simulink model "EV_Model_acc"  (R2024b)
settings: Solver=ode23tb  StartTime=0  StopTime=195  RelTol=1e-3
undefined symbols (not defined in the file): Battery, BattSocInit, DiscIntNeverNeededParam, disk_abore, MotSpd, MotTrq, mu_kinetic, Ndiff, Np_Module, Ns_Module, num_pads, NumModules, RegenBrkCutOff, RegenBrkSpd_bpt, Rm
libraries: autolibshared x6, autolibsharedcoupling x3, simulink x3, mpcadaslib x1, autolibdatasheetbattery x1, autolibmappedmotor x1, autolibshareddiff x1, SignalEditorBlockLib x1
(part 1 of 3)
settings Model: SimulationMode=accelerator  Creator=mmdvn  LastModifiedBy=r
settings DebuggingCC: AlgebraicLoopMsg=none  ParameterPrecisionLossMsg=none  AllowSymbolicDim=off
settings RTWCC: GPUComputeCapability=3.5

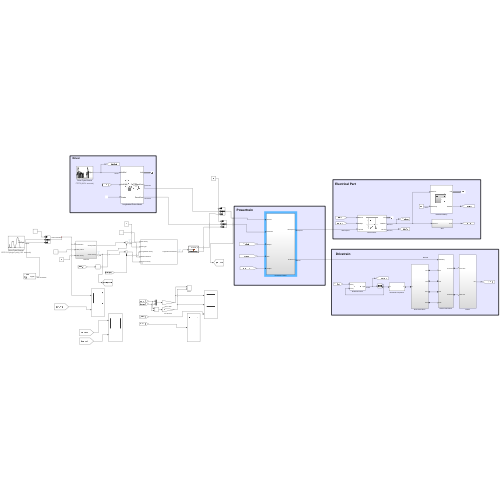
[thumbnail: Simulink's stored preview of the top-level diagram]
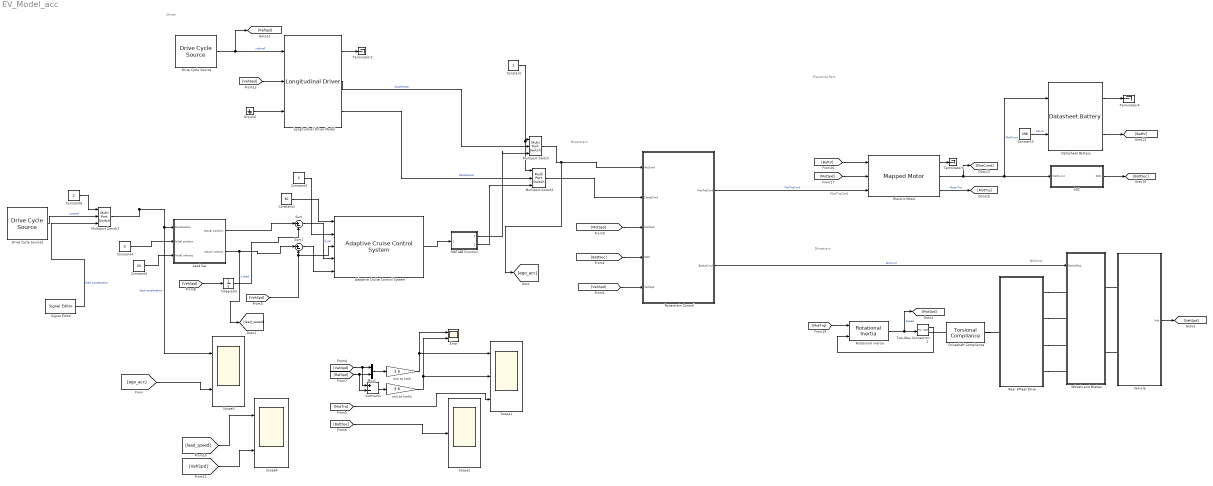
== system EV_Model_acc ==
  note: BrkCmd
  note: MotTrqCmd
  note: Drivetrain
  note: Electrical Part
  note: Powertrain
  note: Driver
  Adaptive Cruise Control System : mpcadaslib/Adaptive Cruise Control System  EgoModel=tf(1,[0.5,1,0])  InitialEgoVelocity=20  DefaultSpacing=10  MaxVelocity=50  MinAcceleration=-3  amin_ext=off  MaxAcceleration=2  amax_ext=off  Ts=0.1  PredictionHorizon=30  ControllerBehavior=0.5  suboptimal=off  maxiter=10  datatypeopt=double  optmode=off  trackmode=off
      settings: LibrarySourceBlock=mpclib/Automated Driving/Adaptive Cruise Control System
  Constant : Constant  Value=2
  Constant1 : Constant  Value=30
  Constant2 : Constant  Value=2
  Constant3 : Constant  Value=298
  Constant4 : Constant  Value=0
  Constant5 : Constant  Value=20
  Constant6 : Constant  Value=2
  Datasheet Battery : autolibdatasheetbattery/Datasheet Battery  CapacityCtrl=Parameter  OutputVlt=Unfiltered  BattChargeMax=5  Em=[2.8 3.228 3.284 3.361 3.408 3.427 3.472 3.477 3.493 3.504 3.516 3.528 3.537 3.545 3.555 3.561 3.566 3.576 3.587 3.589 3.594 3.6 3.608 3.61 3.616 3.619 3.626 3.632 3.637 3.64 3.645 3.646 3.652 3.655 3.658 3.661 3.664 3.668 3.673 3.678 3.68 3.681 3.686 3.692 3.699 3.702 3.705 3.71 3.717 3.723 3.728 3.733 3.735 3.742 3.749 3.755 3.761 3.768 3.773 3.78 3.791 3.798 3.798 3.814 3.818 3.825 3.841 3.846 3.855 3.863 3.877 3.885 3.894 3.907 3.919 3.926 3.935 3.944 3.954 3.964 3.974 3.988 3.998 4.014 4.029 4.034 4.047 4.065 4.074 4.086 4.097 4.131 4.126 4.138 4.15 4.18 4.174 4.187 4.207 4.231 4.221]  CapLUTBp=[0 0.01 0.02 0.03 0.04 0.05 0.06 0.07 0.08 0.09 0.1 0.11 0.12 0.13 0.14 0.15 0.16 0.17 0.18 0.19 0.2 0.21 0.22 0.23 0.24 0.25 0.26 0.27 0.28 0.29 0.3 0.31 0.32 0.33 0.34 0.35 0.36 0.37 0.38 0.39 0.4 0.41 0.42 0.43 0.44 0.45 0.46 0.47 0.48 0.49 0.5 0.51 0.52 0.53 0.54 0.55 0.56 0.57 0.58 0.59 0.6 0.61 0.62 0.63 0.64 0.65 0.66 0.67 0.68 0.69 0.7 0.71 0.72 0.73 0.74 0.75 0.76 0.77 0.78 0.79 0.8 0.81 0.82 0.83 0.84 0.85 0.86 0.87 0.88 0.89 0.9 0.91 0.92 0.93 0.94 0.95 0.96 0.97 0.98 0.99 1]  RInt=[0.008846 0.009319 0.009027 0.00847 0.01032 0.01314;0.006389 0.006554 0.005553 0.005525 0.006043 0.007805;0.004364 0.004101 0.00406 0.003452 0.003846 0.004517;0.002031 0.002563 0.002532 0.00246 0.002716 0.003047;0.001443 0.001825 0.001795 0.001778 0.001924 0.002234;0.0005603 0.0007192 0.0006887 0.0007557 0.0007355 0.001014;0.001028 0.001338 0.001 0.001536 0.001546 0.002789]  BattTempBp=[243.1 253.1 263.1 273.1 283.1 298.1 313.1]  CapSOCBp=[0 0.2 0.4 0.6 0.8 1]  Ns=48  Np=31  BattCapInit=3.6  Tc=1/1000  Vinit=4.221  RefBlkName='autolibdatasheetbattery/Datasheet Battery'
  Drive Cycle Source : autolibshared/Drive Cycle Source  cycleVar=FTP75  fileVar=cycleFTP75.mat  tfinal="2474  seconds"  cycleRepeat=off  outAccPort=off  outGearPort=off  gearList=No gear data  t_wot1=5  xdot_woto=0  xdot_wot1=30  t_wot2=20  xdot_wot2=0  t_wotend=30  srcUnit=m/s  outUnit=m/s  srcAccUnit=m/s/s  outAccUnit=m/s^2  dt=0  aMode=1  faultOption=off  velBnd=2  velBndUnit=mph  inUnit=m/s  timeBnd=1  failOption=off  stopSim=off  maxFaultCnt=10  maxFaultTime=2  maxTotFaultTime=15  traceOption=off  dtTrace=1  traceWindow=10  lastDCname=FTP75  lastOutUnit=mph  lastDT=0  lastTB=1  lastSB=2  forceCalcBound=off
  Drive Cycle Source1 : autolibshared/Drive Cycle Source  cycleVar=ECE R15 (single cycle)  fileVar=cycleFTP75.mat  tfinal="195  seconds"  cycleRepeat=off  outAccPort=off  outGearPort=off  gearList=No gear data  t_wot1=5  xdot_woto=0  xdot_wot1=30  t_wot2=20  xdot_wot2=0  t_wotend=30  srcUnit=m/s  outUnit=m/s  srcAccUnit=m/s/s  outAccUnit=m/s^2  dt=0  aMode=1  faultOption=off  velBnd=2  velBndUnit=mph  inUnit=m/s  timeBnd=1  failOption=off  stopSim=off  maxFaultCnt=10  maxFaultTime=2  maxTotFaultTime=15  traceOption=off  dtTrace=1  traceWindow=10  lastDCname=ECE R15 (single cycle)  lastOutUnit=mph  lastDT=0  lastTB=1  lastSB=2  forceCalcBound=off
  Driveshaft Compliance : autolibsharedcoupling/Torsional Compliance  port_config=Two-way connection  extInfo=off  k=10000  b=400  theta_o=0  domega_o=0  omega_c=100  blkID=0  aMode=1
  Electric Motor : autolibmappedmotor/Mapped Motor  w_Tmax_bp_ext=w_Tmax_bp  Tmax_w_V_ext=Tmax_w_V  w_Tmin_bp_ext=w_Tmin_bp  Tmin_w_V_ext=Tmin_w_V  port_config=Speed  param_by=Maximum torque and power  w_t=[ 0 375 750 800 ]  T_t=[0.09 0.08 0.07 0]  torque_max=450  power_max=211000  SpreadsheetTqLimitsFileName=MotorCalibrationImportData.xlsx  Tmax_w_V=[0.09 0.09 0.09;0.08 0.08 0.08;0.07 0.07 0.07;0 0 0]  w_Tmax_bp=[ 0 375 750 800 ]  V_Tmax_bp=[500 750 900]  Tmin_w_V=[-0.09 -0.09 -0.09;-0.08 -0.08 -0.08;-0.07 -0.07 -0.07;0 0 0]  w_Tmin_bp=[ 0 375 750 800 ]  V_Tmin_bp=[500 750 900]  Tc=0.02  param_loss=Tabulated efficiency data  SpreadsheetLossFileName=MotorCalibrationImportData.xlsx  SpreadsheetEffFileName=MotorCalibrationImportData.xlsx  eff=100  w_eff=375  T_eff=0.08  Piron=0  Pbase=0  w_eff_bp=[-800 -400 0 400 800]  T_eff_bp=[0 0.03 0.06 0.09]  Temp_eff_bp=[233.15 293.15 373.15]  V_eff_bp=[500 700 900]  losses_table=[1.49 1.67 2.21 3.10; 0.42 0.69 1.14 2.03; 0.06 0.24 0.78 1.68; 0.42 0.69 1.14 2.03; 1.49 1.67 2.21 3.10]  losses_table_3d=cat(3,[1.49 1.67 2.21 3.10; 0.42 0.69 1.14 2.03; 0.06 0.24 0.78 1.68; 0.42 0.69 1.14 2.03; 1.49 1.67 2.21 3.10],[1.49 1.67 2.21 3.10; 0.42 0.69 1.14 2.03; 0.06 0.24 0.78 1.68; 0.42 0.69 1.14 2.03; 1.49 1.67 2.21 3.10],[1.49 1.67 2.21 3.10; 0.42 0.69 1.14 2.03; 0.06 0.24 0.78 1.68; 0.42 0.69 1.14 2.03; 1.49 1.67 2.21 3.10])  losses_table_4d=cat(4,cat(3,[1.5645 0.441 0.063 0.441 1.5645;1.7535 0.7245 0.252 0.7245 1.7535;2.3205 1.197 0.819 1.197 2.3205;3.255 2.1315 1.764 2.1315 3.255],[1.5645 0.441 0.063 0.441 1.5645;1.7535 0.7245 0.252 0.7245 1.7535;2.3205 1.197 0.819 1.197 2.3205;3.255 2.1315 1.764 2.1315 3.255],[1.5645 0.441 0.063 0.441 1.5645;1.7535 0.7245 0.252 0.7245 1.7535;2.3205 1.197 0.819 1.197 2.3205;3.255 2.1315 1.764 2.1315 3.255]),cat(3,[1.49 0.42 0.06 0.42 1.49;1.67 0.69 0.24 0.69 1.67;2.21 1.14 0.78 1.14 2.21;3.1 2.03 1.68 2.03 3.1],[1.49 0.42 0.06 0.42 1.49;1.67 0.69 0.24 0.69 1.67;2.21 1.14 0.78 1.14 2.21;3.1 2.03 1.68 2.03 3.1],[1.49 0.42 0.06 0.42 1.49;1.67 0.69 0.24 0.69 1.67;2.21 1.14 0.78 1.14 2.21;3.1 2.03 1.68 2.03 3.1]),cat(3,[1.5347 0.4326 0.0618 0.4326 1.5347;1.7201 0.7107 0.2472 0.7107 1.7201;2.2763 1.1742 0.8034 1.1742 2.2763;3.193 2.0909 1.7304 2.0909 3.193],[1.5347 0.4326 0.0618 0.4326 1.5347;1.7201 0.7107 0.2472 0.7107 1.7201;2.2763 1.1742 0.8034 1.1742 2.2763;3.193 2.0909 1.7304 2.0909 3.193],[1.5347 0.4326 0.0618 0.4326 1.5347;1.7201 0.7107 0.2472 0.7107 1.7201;2.2763 1.1742 0.8034 1.1742 2.2763;3.193 2.0909 1.7304 2.0909 3.193]))  efficiency_table=[95 95 95 95; 95 95 95 95; 95 95 95 95; 95 95 95 95; 95 95 95 95]  efficiency_table_3d=cat(3,[95 95 95 95; 95 95 95 95; 95 95 95 95; 95 95 95 95; 95 95 95 95],[95 95 95 95; 95 95 95 95; 95 95 95 95; 95 95 95 95; 95 95 95 95],[95 95 95 95; 95 95 95 95; 95 95 95 95; 95 95 95 95; 95 95 95 95])  efficiency_table_4d=cat(4,cat(3,90*ones(5,4)',90*ones(5,4)',90*ones(5,4)'),cat(3,95*ones(5,4)',95*ones(5,4)',95*ones(5,4)'),cat(3,92*ones(5,4)',92*ones(5,4)',92*ones(5,4)'))  J=5e-6  b=1e-5  omega_o=0  T_t_extended=[0 0.07 0.08 0.09 0.08 0.07 0]  w_t_extended=[-800 -750 -375 0 375 750 800]  KLossIron=0  KLossCopper=0  x_w_eff_vec=[-800 -400 0 400 800]  x_T_eff_vec=[-0.09 -0.06 -0.03 0 0.03 0.06 0.09]  x_tmp_eff_vec=[-0.09 -0.06 -0.03 0 0.03 0.06 0.09]  x_V_eff_vec=[500 700 900]  x_losses_mat=[3.78947368421052 2.52631578947368 1.26315789473684 0 1.2 2.4 3.6;1.89473684210526 1.26315789473684 0.63157894736842 0 0.599999999999999 1.2 1.8;0 0 0 0 0 0 0;1.8 1.2 0.599999999999999 0 0.63157894736842 1.26315789473684 1.89473684210526;3.6 2.4 1.2 0 1.26315789473684 2.52631578947368 3.78947368421052]  x_losses_mat_3d=[37.8947368421052 25.2631578947368 12.6315789473684 0 12 24 36;18.9473684210526 12.6315789473684 6.3157894736842 0 5.99999999999999 12 18;0 0 0 0 0 0 0;18 12 5.99999999999999 0 6.3157894736842 12.6315789473684 18.9473684210526;36 24 12 0 12.6315789473684 25.2631578947368 37.8947368421052]  x_losses_mat_4d=cat(4,cat(3,[1.5645 0.441 0.063 0.441 1.5645;1.7535 0.7245 0.252 0.7245 1.7535;2.3205 1.197 0.819 1.197 2.3205;3.255 2.1315 1.764 2.1315 3.255],[1.5645 0.441 0.063 0.441 1.5645;1.7535 0.7245 0.252 0.7245 1.7535;2.3205 1.197 0.819 1.197 2.3205;3.255 2.1315 1.764 2.1315 3.255],[1.5645 0.441 0.063 0.441 1.5645;1.7535 0.7245 0.252 0.7245 1.7535;2.3205 1.197 0.819 1.197 2.3205;3.255 2.1315 1.764 2.1315 3.255]),cat(3,[1.49 0.42 0.06 0.42 1.49;1.67 0.69 0.24 0.69 1.67;2.21 1.14 0.78 1.14 2.21;3.1 2.03 1.68 2.03 3.1],[1.49 0.42 0.06 0.42 1.49;1.67 0.69 0.24 0.69 1.67;2.21 1.14 0.78 1.14 2.21;3.1 2.03 1.68 2.03 3.1],[1.49 0.42 0.06 0.42 1.49;1.67 0.69 0.24 0.69 1.67;2.21 1.14 0.78 1.14 2.21;3.1 2.03 1.68 2.03 3.1]),cat(3,[1.5347 0.4326 0.0618 0.4326 1.5347;1.7201 0.7107 0.2472 0.7107 1.7201;2.2763 1.1742 0.8034 1.1742 2.2763;3.193 2.0909 1.7304 2.0909 3.193],[1.5347 0.4326 0.0618 0.4326 1.5347;1.7201 0.7107 0.2472 0.7107 1.7201;2.2763 1.1742 0.8034 1.1742 2.2763;3.193 2.0909 1.7304 2.0909 3.193],[1.5347 0.4326 0.0618 0.4326 1.5347;1.7201 0.7107 0.2472 0.7107 1.7201;2.2763 1.1742 0.8034 1.1742 2.2763;3.193 2.0909 1.7304 2.0909 3.193]))  CalLossMapData={}  CalLossWithTempMapData={}  aMode=1  RefBlkName='autolibmappedmotor/Mapped Motor'
      settings: LibrarySourceBlock=autolibemachines/Mapped Motor
  Error : Scope  NumInputPorts=2
  Ground : Ground
  Integrator : Integrator
  Lead Car : Subsystem
  Longitudinal Driver Model : autolibshared/Longitudinal Driver  extAccelOvr=off  extDecelOvr=off  extAccelHld=off  extDecelHld=off  extAccelZero=off  extDecelZero=off  cntrlType=Predictive  shftType=Reverse, Neutral, Drive  velUnits=m/s  gearOut=off  Kp=1  Ki=1  Kff=0  Kg=0  VehVelVec=[0 100]  KffVec=[.1 .1]  KpVec=[10 10]  KiVec=[5 5]  KgVec=[0 0]  m=1645  Kpt=450*9.04/0.324  tau=0.12  L=4  aR=30.3/3875  bR=0.21290*4.44822/0.44704  cR=0.01278*4.44822/0.44704^2  g=9.81  vnom=1  Kaw=0  tauerr=0  tauPt=2  GearInit=0  tShift=.1  pdlVec=[0.1 0.4 0.5 0.9]  upShftTbl=[-1 12.9375 26.4375 39.9375 51.18749999999999 62.4375 72.84375 83.25;-1 16.3125 29.8125 43.3125 54.5624 65.8125 76.78125 87.75;-1 19.6875 33.1875 46.68749999999999 57.9375 69.1875 80.71875 92.25;-1 33 52.5 77.25 100.5 138.75 161.875 185]  dwnShftTbl=[1 9.5625 23.0625 36.5625 47.8125 59.0625 68.90625 78.75;1 12.9375 26.4375 39.9375 51.18749999999999 62.4375 72.84375 83.25;1 16.3125 29.8125 43.3125 54.562499 65.8125 76.78125 87.75;1 19.6875 33.1875 46.68749999999999 57.9375 69.1875 80.71875 92.25]  tClutch=.5  tRev=.5  tPark=120  aMode=1  UpGearVec="[0  1  2  3  4  5  6  7]"  DownGearVec="[1  2  3  4  5  6  7  8]"
  MATLAB Function : MATLAB Function  TreatAsAtomicUnit=on
  Multiport Switch : MultiPortSwitch  Inputs=2  SaturateOnIntegerOverflow=off  InputSameDT=off
  Multiport Switch1 : MultiPortSwitch  Inputs=2  SaturateOnIntegerOverflow=off  InputSameDT=off
  Multiport Switch2 : MultiPortSwitch  Inputs=2  SaturateOnIntegerOverflow=off  InputSameDT=off
  Mux1 : Mux  Inputs=2
  Powertrain Control : Subsystem
  Rear Wheel Drive : Subsystem  VariantControl=1
  "Rotational Inertia " : autolibsharedcoupling/Rotational Inertia  port_config=Simulink  extInfo=off  externJ=off  J=0.1  b=.001  omega_o=0  blkID=0  aMode=1
      settings: LibrarySourceBlock=autolibcoupling/Rotational Inertia
  SOC : Subsystem
  Scope1 : Scope  NumInputPorts=3
  Scope2 : Scope
  Scope3 : Scope  NumInputPorts=2
  Scope4 : Scope  NumInputPorts=2
  Signal Editor : SignalEditorBlockLib/Signal Editor  FileName=cycle.mat  ActiveScenario=Scenario  ActiveSignal=Signal 1  IsBus=off  OutputBusObjectStr=Bus: BusObject  SampleTime=0  Interpolate=off  ZeroCross=off  OutputAfterFinalValue=Setting to zero  Unit=inherit  PreserveSignalName=on  ApplySigPropsToAllScenarios=on  ApplySigPropsToAllSignals=off
  Subtract1 : Sum  Inputs=+-
  Sum : Sum  Inputs=|+-
  Sum1 : Sum  Inputs=|+-
  Terminator2 : Terminator
  Terminator3 : Terminator
  Terminator4 : Terminator
  Two-Way Connection1 : TwoWayConnection
  Vehicle : Subsystem
  Wheels and Brakes : Subsystem  VariantControl=0
  m/s to kmh : Gain  Gain=3.6
  m/s to kmh1 : Gain  Gain=3.6
  wires:
  Two-Way Connection1/1 -> "Rotational Inertia "/2
  Vehicle/1(Info) -> [VehSpd]
  [MotSpd] -> Powertrain Control/3(MotSpd)
  [BattSoc] -> Powertrain Control/4(SOC)
  Powertrain Control/1(MotTrqCmd) -> Electric Motor/3  "MotTrqCmd"
  Powertrain Control/2(BrakeCmd) -> Wheels and Brakes/1(BrakeReq)  "BrkCmd"
  Drive Cycle Source/1 -> Longitudinal Driver Model/1, [RefSpd]  "xdotref"
  Ground/1 -> Longitudinal Driver Model/3
  [VehSpd] -> Longitudinal Driver Model/2
  "Rotational Inertia "/1 -> [MotSpd], Two-Way Connection1/1  "Speed"
  Longitudinal Driver Model/2 -> Multiport Switch/2  "Accelerator"
  Longitudinal Driver Model/1 -> Terminator2/1
  [MotTrq] -> "Rotational Inertia "/1
  Constant3/1 -> Datasheet Battery/2  "Kelvin"
  [MotSpd] -> Electric Motor/2
  Datasheet Battery/1 -> Terminator4/1
  Datasheet Battery/2 -> [BattV]
  Electric Motor/3 -> [MotTrq]  "MotorTrq"
  Electric Motor/2 -> Datasheet Battery/1, SOC/1(MotCurnt), [MotCurnt]  "MotCurnt"
  Electric Motor/1 -> Terminator3/1
  SOC/1(SOC) -> [BattSoc]
  [VehSpd] -> Powertrain Control/5(VehSpd)
  [BattV] -> Electric Motor/1
  [MotTrq] -> Scope1/3
  m/s to kmh/1 -> Error/1, Scope1/1
  [RefSpd] -> Subtract1/2, Mux1/2
  [VehSpd] -> Subtract1/1, Mux1/1
  Mux1/1 -> m/s to kmh/1
  Subtract1/1 -> m/s to kmh1/1
  m/s to kmh1/1 -> Error/2, Scope1/2
  [BattSoc] -> Scope2/1
  Lead Car/1(Actual position) -> Sum/1
  Lead Car/2(Actual velocity) -> [lead_speed], Sum1/1  "v_lead"
  [VehSpd] -> Integrator/1
  [VehSpd] -> Adaptive Cruise Control System/3, Sum1/2
  Sum1/1 -> Adaptive Cruise Control System/5
  Sum/1 -> Adaptive Cruise Control System/4  "d_rel"
  Integrator/1 -> Sum/2
  Multiport Switch/1 -> [ego_acc], Powertrain Control/1(AccCmd)
  Constant/1 -> Multiport Switch1/1, Multiport Switch/1
  Adaptive Cruise Control System/1 -> MATLAB Function/1(a_desired)
  MATLAB Function/1(AccelPID_In) -> Multiport Switch/3
  Longitudinal Driver Model/3 -> Multiport Switch1/2  "Decelerator"
  Multiport Switch1/1 -> Powertrain Control/2(DecelCmd)
  MATLAB Function/2(BrakePID_In) -> Multiport Switch1/3
  Constant1/1 -> Adaptive Cruise Control System/1
  Constant2/1 -> Adaptive Cruise Control System/2
  Multiport Switch2/1 -> Scope3/1, Lead Car/1(Acceleration)  "lead acceleration"
  Constant5/1 -> Lead Car/3(Initial velocity)
  Constant4/1 -> Lead Car/2(Initial position)
  [ego_acc] -> Scope3/2
  [lead_speed] -> Scope4/1
  [VehSpd] -> Scope4/2
  Drive Cycle Source1/1 -> Multiport Switch2/2  "xdotref"
  Signal Editor/1 -> Multiport Switch2/3  "lead acceleration"
  Constant6/1 -> Multiport Switch2/1
  connections:
  Rear Wheel Drive/RConn3 -- Wheels and Brakes/LConn3
  Rear Wheel Drive/RConn4 -- Wheels and Brakes/LConn4
  Driveshaft Compliance/LConn1 -- Two-Way Connection1/RConn1
  Rear Wheel Drive/RConn1 -- Wheels and Brakes/LConn1
  Rear Wheel Drive/RConn2 -- Wheels and Brakes/LConn2
  Vehicle/LConn1 -- Wheels and Brakes/RConn1
  Vehicle/LConn2 -- Wheels and Brakes/RConn2
  Driveshaft Compliance/RConn1 -- Rear Wheel Drive/LConn1

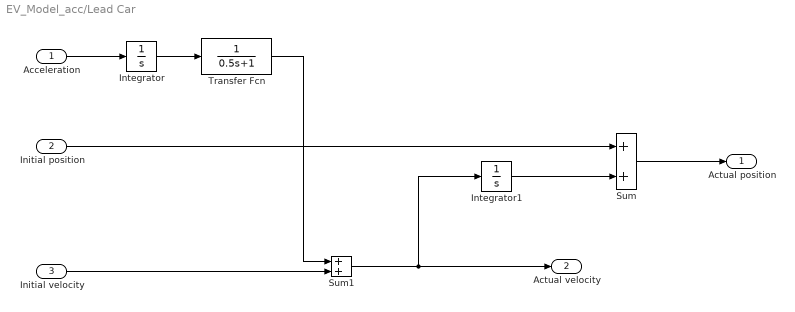
== system EV_Model_acc/Lead Car ==
  Acceleration : Inport
  Initial position : Inport  Port=2
  Initial velocity : Inport  Port=3
  Integrator : Integrator
  Integrator1 : Integrator
  Sum : Sum
  Sum1 : Sum
  Transfer Fcn : TransferFcn  Denominator=[0.5 1]
  Actual position : Outport  VectorParamsAs1DForOutWhenUnconnected=off
  Actual velocity : Outport  Port=2  VectorParamsAs1DForOutWhenUnconnected=off
  wires:
  Transfer Fcn/1 -> Sum1/1
  Initial velocity/1 -> Sum1/2
  Sum/1 -> Actual position/1
  Integrator/1 -> Transfer Fcn/1
  Sum1/1 -> Integrator1/1, Actual velocity/1
  Acceleration/1 -> Integrator/1
  Initial position/1 -> Sum/1
  Integrator1/1 -> Sum/2

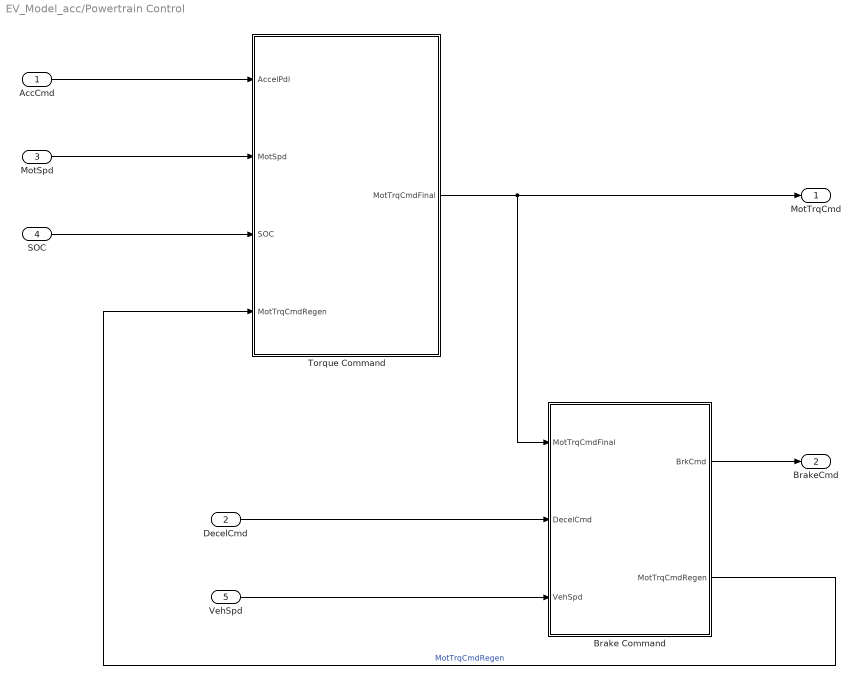
== system EV_Model_acc/Powertrain Control ==
  AccCmd : Inport
  DecelCmd : Inport  Port=2  OutDataTypeStr=double
  MotSpd : Inport  Port=3
  SOC : Inport  Port=4
  VehSpd : Inport  Port=5
  Brake Command : Subsystem  InitFcn=%[~]=autosharedicon('autolibutils',gcb,0);  VariantControl=Variant
  Torque Command : Subsystem
  MotTrqCmd : Outport  VectorParamsAs1DForOutWhenUnconnected=off
  BrakeCmd : Outport  Port=2  VectorParamsAs1DForOutWhenUnconnected=off
  wires:
  SOC/1 -> Torque Command/3(SOC)
  MotSpd/1 -> Torque Command/2(MotSpd)
  DecelCmd/1 -> Brake Command/2("DecelCmd ")
  AccCmd/1 -> Torque Command/1(AccelPdl)
  Torque Command/1(MotTrqCmdFinal) -> MotTrqCmd/1, Brake Command/1(MotTrqCmdFinal)
  Brake Command/1(" BrkCmd") -> BrakeCmd/1
  VehSpd/1 -> Brake Command/3(VehSpd)
  Brake Command/2(" MotTrqCmdRegen") -> Torque Command/4(MotTrqCmdRegen)  "MotTrqCmdRegen"

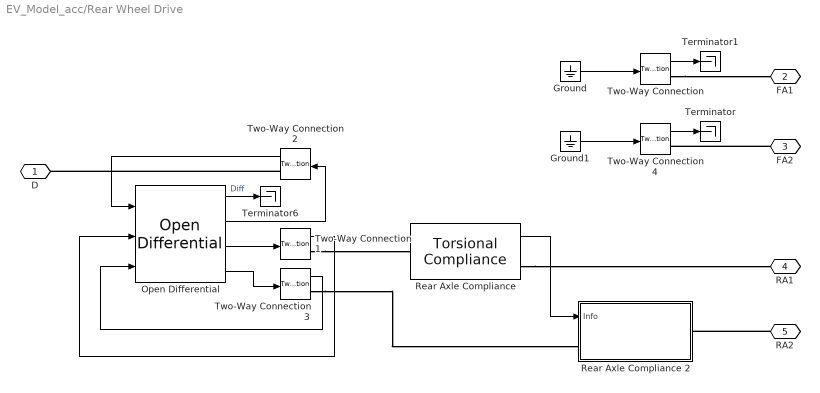
== system EV_Model_acc/Rear Wheel Drive ==
  Ground : Ground
  Ground1 : Ground
  "Open Differential " : autolibshareddiff/Open Differential  DiffEffModelPopup=Constant  InterpMethod=Linear point-slope  extTamb=off  shaftSwitchMask=To the left of center-line  Ndiff=Ndiff  Jd=0.025  bd=0.001  Jw1=0.01  bw1=0.001  Jw2=0.01  bw2=0.001  omegaw1o=0  omegaw2o=0  eta=1  eta_tbl=reshape([0.64 0.76 0.8 0.81 0.83 0.84 0.84 0.56 0.73 0.78 0.8 0.83 0.84 0.84 0.54 0.71 0.77 0.8 0.82 0.84 0.84 0.53 0.71 0.77 0.8 0.83 0.84 0.84 0.51 0.71 0.77 0.8 0.83 0.84 0.85 0.52 0.7 0.77 0.8 0.83 0.84 0.85 0.51 0.71 0.76 0.79 0.83 0.84 0.85 0.5 0.69 0.76 0.79 0.82 0.84 0.85 0.45 0.68 0.75 0.78 0.82 0.84 0.85 0.43 0.67 0.74 0.78 0.81 0.83 0.84 0.38 0.63 0.71 0.75 0.8 0.82 0.83 0.81 0.86 0.88 0.89 0.89 0.89 0.9 0.77 0.85 0.87 0.88 0.89 0.9 0.9 0.72 0.82 0.86 0.87 0.88 0.89 0.9 0.68 0.8 0.84 0.86 0.88 0.89 0.89 0.67 0.8 0.84 0.86 0.88 0.89 0.9 0.67 0.8 0.84 0.86 0.88 0.89 0.9 0.65 0.8 0.84 0.86 0.88 0.89 0.9 0.64 0.79 0.83 0.86 0.88 0.89 0.9 0.63 0.78 0.83 0.86 0.88 0.89 0.9 0.59 0.76 0.82 0.85 0.87 0.89 0.9 0.53 0.73 0.8 0.83 0.86 0.88 0.89], 7, 11, 2)  Trq_bpts=[25, 50, 75, 100, 150, 200, 250]  omega_bpts=[52.4 78.5 105 131 157 183 209 262 314 419 524]  Temp_bpts=[290 358]  Tamb=297.15  maxAbsSpd=5e3  aMode=1
      settings: LibrarySourceBlock=autolibdiff/Open Differential
  Rear Axle Compliance : autolibsharedcoupling/Torsional Compliance  port_config=Two-way connection  extInfo=on  k=10000  b=400  theta_o=0  domega_o=0  omega_c=100  blkID=0  aMode=1
  Rear Axle Compliance 2 : Subsystem
  Terminator : Terminator
  Terminator1 : Terminator
  Terminator6 : Terminator
  Two-Way Connection{,1..4} (5 alike) : TwoWayConnection
  D : PMIOPort  Side=Left
  FA1 : PMIOPort  Port=2  Side=Right
  FA2 : PMIOPort  Port=3  Side=Right
  RA1 : PMIOPort  Port=4  Side=Right
  RA2 : PMIOPort  Port=5  Side=Right
  wires:
  Two-Way Connection3/1 -> "Open Differential "/3
  "Open Differential "/4 -> Two-Way Connection3/1
  "Open Differential "/2 -> Two-Way Connection2/1
  Two-Way Connection1/1 -> "Open Differential "/2
  Two-Way Connection2/1 -> "Open Differential "/1
  "Open Differential "/1 -> Terminator6/1  "Diff"
  "Open Differential "/3 -> Two-Way Connection1/1
  Rear Axle Compliance/1 -> Rear Axle Compliance 2/1(Info)
  Two-Way Connection/1 -> Terminator1/1
  Ground/1 -> Two-Way Connection/1
  Ground1/1 -> Two-Way Connection4/1
  Two-Way Connection4/1 -> Terminator/1
  connections:
  Two-Way Connection1/RConn1 -- Rear Axle Compliance/LConn1
  Two-Way Connection3/RConn1 -- Rear Axle Compliance 2/LConn1
  Two-Way Connection2/RConn1 -- D/RConn1
  Rear Axle Compliance/RConn1 -- RA1/RConn1
  RA2/RConn1 -- Rear Axle Compliance 2/RConn1
  Two-Way Connection/RConn1 -- FA1/RConn1
  FA2/RConn1 -- Two-Way Connection4/RConn1

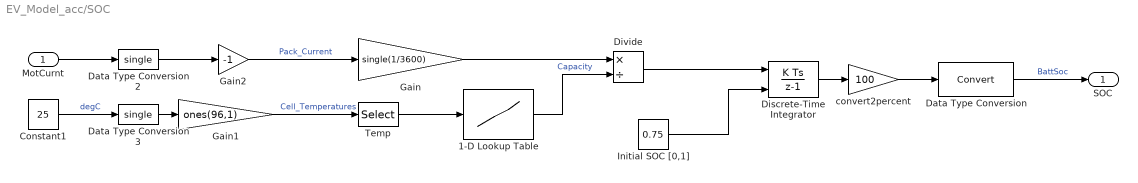
== system EV_Model_acc/SOC ==
  MotCurnt : Inport  PortDimensions=1
  1-D Lookup Table : Lookup_n-D  NumberOfTableDimensions=1  BreakpointsForDimension1=single(Battery.Temperature_LUT)  Table=single(Battery.Capacity_LUT)*Np_Module  InternalRulePriority=Speed  RndMeth=Simplest
  Constant1 : Constant  Value=25
  Data Type Conversion : DataTypeConversion  SaturateOnIntegerOverflow=off  RndMeth=Floor
  Data Type Conversion2 : DataTypeConversion  OutDataTypeStr=single  SaturateOnIntegerOverflow=off  RndMeth=Floor
  Data Type Conversion3 : DataTypeConversion  OutDataTypeStr=single  SaturateOnIntegerOverflow=off  RndMeth=Floor
  Discrete-Time Integrator : DiscreteIntegrator  InitialConditionSource=external  InitialCondition=single(BattSocInit)  SampleTime=-1  LimitOutput=on  UpperSaturationLimit=1  LowerSaturationLimit=0  ICPrevOutput=DiscIntNeverNeededParam  ICPrevScaledInput=DiscIntNeverNeededParam
  Divide : Product  Inputs=*/
  Gain : Gain  Gain=single(1/3600)
  Gain1 : Gain  Gain=ones(96,1)
  Gain2 : Gain  Gain=-1
  Initial SOC [0,1] : Constant  Value=0.75  OutDataTypeStr=single
  Temp : Selector  InputPortWidth=Ns_Module*NumModules  IndexOptions=Index vector (dialog)  Indices=1  OutputSizes=1
  convert2percent : Gain  Gain=100
  SOC : Outport
  wires:
  Gain1/1 -> Temp/1  "Cell_Temperatures"
  Gain2/1 -> Gain/1  "Pack_Current"
  Data Type Conversion2/1 -> Gain2/1
  Data Type Conversion3/1 -> Gain1/1
  MotCurnt/1 -> Data Type Conversion2/1
  Constant1/1 -> Data Type Conversion3/1  "degC"
  convert2percent/1 -> Data Type Conversion/1
  Data Type Conversion/1 -> SOC/1  "BattSoc"
  Discrete-Time Integrator/1 -> convert2percent/1
  Temp/1 -> 1-D Lookup Table/1
  Divide/1 -> Discrete-Time Integrator/1
  1-D Lookup Table/1 -> Divide/2  "Capacity"
  Gain/1 -> Divide/1
  Initial SOC [0,1]/1 -> Discrete-Time Integrator/2

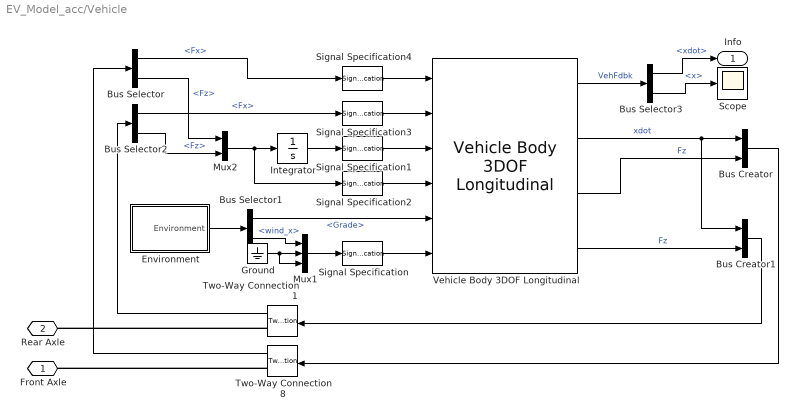
== system EV_Model_acc/Vehicle ==
  Bus Creator : BusCreator  Inputs=2
  Bus Creator1 : BusCreator  Inputs=2
  Bus Selector : BusSelector  OutputSignals=Fx,Fz
  Bus Selector1 : BusSelector  OutputSignals=Ground.Grade,Wind.wind_x
  Bus Selector2 : BusSelector  OutputSignals=Fx,Fz
  Bus Selector3 : BusSelector  OutputSignals=BdyFrm.Cg.Vel.xdot,BdyFrm.Cg.Disp.x
  Environment : Subsystem
      mask Display: disp(getString(message('autoblks:autoblkVehMask:environ')))
  Ground : Ground
  Integrator : Integrator
  Mux1 : Mux  Inputs=3
  Mux2 : Mux  Inputs=2
  Scope : Scope
  Signal Specification : SignalSpecification  Unit=m/s
  Signal Specification1 : SignalSpecification  Unit=m
  Signal Specification2 : SignalSpecification  Unit=m/s
  Signal Specification3 : SignalSpecification  Unit=N
  Signal Specification4 : SignalSpecification  Unit=N
  Two-Way Connection1 : TwoWayConnection
  Two-Way Connection8 : TwoWayConnection
  Vehicle Body 3DOF Longitudinal : autolibshared/Vehicle Body 3DOF Longitudinal  VariantControl=SL  groundType=Axle displacement, velocity  aMode=1  extFMode=off  extMMode=off  extTamb=off  NF=2  NR=2  m=1200  a=1.4  b=1.8  h=.35  Cd=.3  Af=2  x_o=0  xdot_o=0  Cl=.1  z_o=-.35  zdot_o=0  Iyy=3500  Cpm=.1  theta_o=0  q_o=0  FskF=[-50, -1, 0, 2, 3, 52].*1.5e4  dzsF=[-5e-3, -1e-4, 0, .2, .2001, .2051]  FsbF=[-10000 -100 -10 0 10 100 10000]  dzdotsF=[-10 -1 -.1 0 .1 1 10]  FskR=[-50, -1, 0, 2, 3, 52].*1e4  dzsR=[-5e-3, -1e-4, 0, .2, .2001, .2051]  FsbR=[-10000 -100 -10 0 10 100 10000]  dzdotsR=[-10 -1 -.1 0 .1 1 10]  Pabs=101325  T=273  g=9.81  blkID=0
      settings: LibrarySourceBlock=autolibvehdynlong/Vehicle Body 3DOF Longitudinal
  Front Axle : PMIOPort  Side=Left
  Rear Axle : PMIOPort  Port=2  Side=Left
  Info : Outport  VectorParamsAs1DForOutWhenUnconnected=off
  wires:
  Vehicle Body 3DOF Longitudinal/3 -> Bus Creator/2  "Fz"
  Vehicle Body 3DOF Longitudinal/2 -> Bus Creator1/1, Bus Creator/1  "xdot"
  Two-Way Connection8/1 -> Bus Selector/1
  Ground/1 -> Mux1/2, Mux1/3
  Mux1/1 -> Signal Specification/1
  Vehicle Body 3DOF Longitudinal/4 -> Bus Creator1/2  "Fz"
  Mux2/1 -> Integrator/1, Signal Specification2/1
  Integrator/1 -> Signal Specification1/1
  Bus Selector1/1 -> Vehicle Body 3DOF Longitudinal/5  "<Grade>"
  Signal Specification/1 -> Vehicle Body 3DOF Longitudinal/6
  Signal Specification1/1 -> Vehicle Body 3DOF Longitudinal/3
  Signal Specification2/1 -> Vehicle Body 3DOF Longitudinal/4
  Signal Specification3/1 -> Vehicle Body 3DOF Longitudinal/2
  Signal Specification4/1 -> Vehicle Body 3DOF Longitudinal/1
  Bus Creator/1 -> Two-Way Connection8/1
  Bus Creator1/1 -> Two-Way Connection1/1
  Bus Selector/1 -> Signal Specification4/1  "<Fx>"
  Bus Selector/2 -> Mux2/1  "<Fz>"
  Bus Selector2/1 -> Signal Specification3/1  "<Fx>"
  Bus Selector2/2 -> Mux2/2  "<Fz>"
  Two-Way Connection1/1 -> Bus Selector2/1
  Environment/1(Environment) -> Bus Selector1/1
  Bus Selector1/2 -> Mux1/1  "<wind_x>"
  Bus Selector3/1 -> Info/1  "<xdot>"
  Vehicle Body 3DOF Longitudinal/1 -> Bus Selector3/1  "VehFdbk"
  Bus Selector3/2 -> Scope/1  "<x>"
  connections:
  Two-Way Connection8/RConn1 -- Front Axle/RConn1
  Two-Way Connection1/RConn1 -- Rear Axle/RConn1
